simulink model "Ardupilot_PID_4"  (R2022a)
settings: Solver=VariableStepAuto  StartTime=0.0  StopTime=20.0  RelTol=1e-3
InitFcn:
  | addpath([pwd '/../Modeling']);
undefined symbols (not defined in the file or in its folder): DiscIntNeverNeededParam
libraries: simulink x8
settings Model: Creator=rodri  LastModifiedBy=rodri

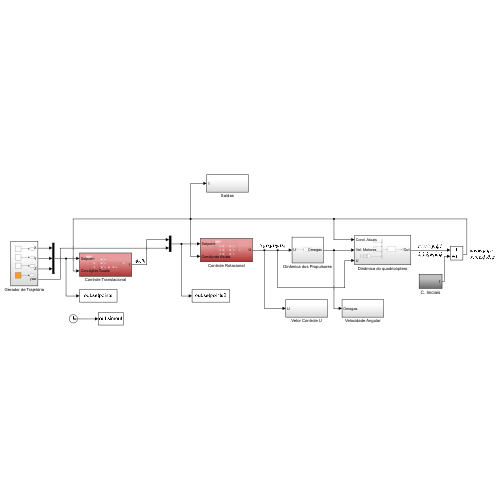
[thumbnail: Simulink's stored preview of the top-level diagram]
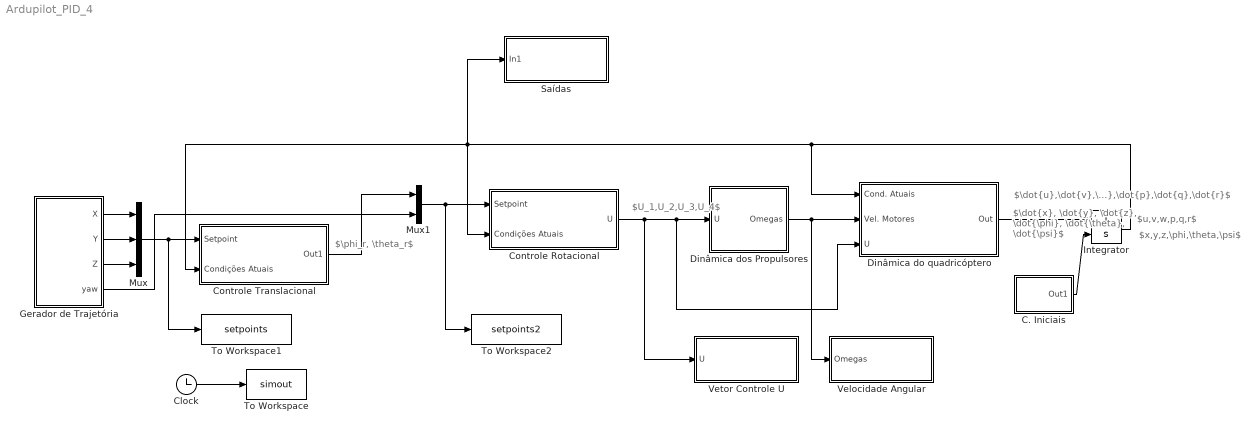
== system Ardupilot_PID_4 ==
  note: $x,y,z,\phi,\theta,\psi$
  note: $U_1,U_2,U_3,U_4$
  note: $u,v,w,p,q,r$
  note: $\phi_r, \theta_r$
  note: $\dot{u},\dot{v},\dot{w},\dot{p},\dot{q},\dot{r}$
  note: $\dot{x}, \dot{y}, \dot{z}, \dot{\phi}, \dot{\theta}, \dot{\psi}$
  C. Iniciais : Subsystem
  Clock : Clock
  Controle Rotacional : Subsystem
  Controle Translacional : Subsystem
  Dinâmica do quadricóptero : Subsystem
  Dinâmica dos Propulsores : Subsystem
  Gerador de Trajetória : Subsystem
  Integrator : Integrator  InitialConditionSource=external
  Mux : Mux  Inputs=3
  Mux1 : Mux  Inputs=2
  Saídas : Subsystem
  To Workspace : ToWorkspace  VariableName=simout  SaveFormat=Structure  SampleTime=-1
  To Workspace1 : ToWorkspace  VariableName=setpoints  SaveFormat=Timeseries  SampleTime=-1
  To Workspace2 : ToWorkspace  VariableName=setpoints2  SaveFormat=Timeseries  SampleTime=-1
  Velocidade Angular : Subsystem
  Vetor Controle U : Subsystem
  wires:
  Integrator/1 -> Dinâmica do quadricóptero/1(Cond. Atuais), Controle Rotacional/2(Condições Atuais), Saídas/1(In1), Controle Translacional/2(Condições Atuais)
  Dinâmica dos Propulsores/1(Omegas) -> Velocidade Angular/1(Omegas), Dinâmica do quadricóptero/2(Vel. Motores)
  Clock/1 -> To Workspace/1
  Controle Rotacional/1(U) -> Dinâmica do quadricóptero/3(U), Dinâmica dos Propulsores/1(U), Vetor Controle U/1(U)
  Mux/1 -> Controle Translacional/1(Setpoint), To Workspace1/1
  Dinâmica do quadricóptero/1(Out) -> Integrator/1
  Gerador de Trajetória/2(Y) -> Mux/2
  Controle Translacional/1(Out1) -> Mux1/1
  Gerador de Trajetória/3(Z) -> Mux/3
  Gerador de Trajetória/4(yaw) -> Mux1/2
  Mux1/1 -> To Workspace2/1, Controle Rotacional/1(Setpoint)
  Gerador de Trajetória/1(X) -> Mux/1
  C. Iniciais/1(Out1) -> Integrator/2

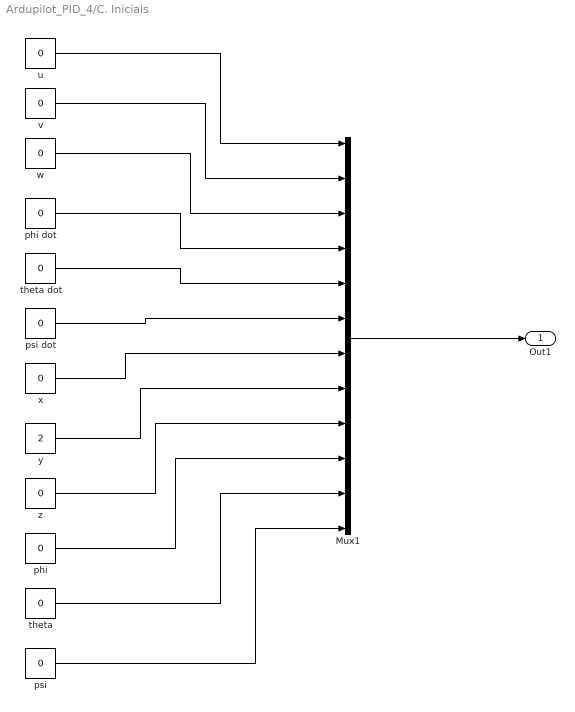
== system Ardupilot_PID_4/C. Iniciais ==
  Mux1 : Mux  Inputs=12
  phi : Constant  Value=0
  phi dot : Constant  Value=0
  psi : Constant  Value=0
  psi dot : Constant  Value=0
  theta : Constant  Value=0
  theta dot : Constant  Value=0
  u : Constant  Value=0
  v : Constant  Value=0
  w : Constant  Value=0
  x : Constant  Value=0
  y : Constant  Value=2
  z : Constant  Value=0
  Out1 : Outport
  wires:
  u/1 -> Mux1/1
  v/1 -> Mux1/2
  w/1 -> Mux1/3
  phi dot/1 -> Mux1/4
  theta dot/1 -> Mux1/5
  psi dot/1 -> Mux1/6
  x/1 -> Mux1/7
  y/1 -> Mux1/8
  z/1 -> Mux1/9
  phi/1 -> Mux1/10
  theta/1 -> Mux1/11
  psi/1 -> Mux1/12
  Mux1/1 -> Out1/1

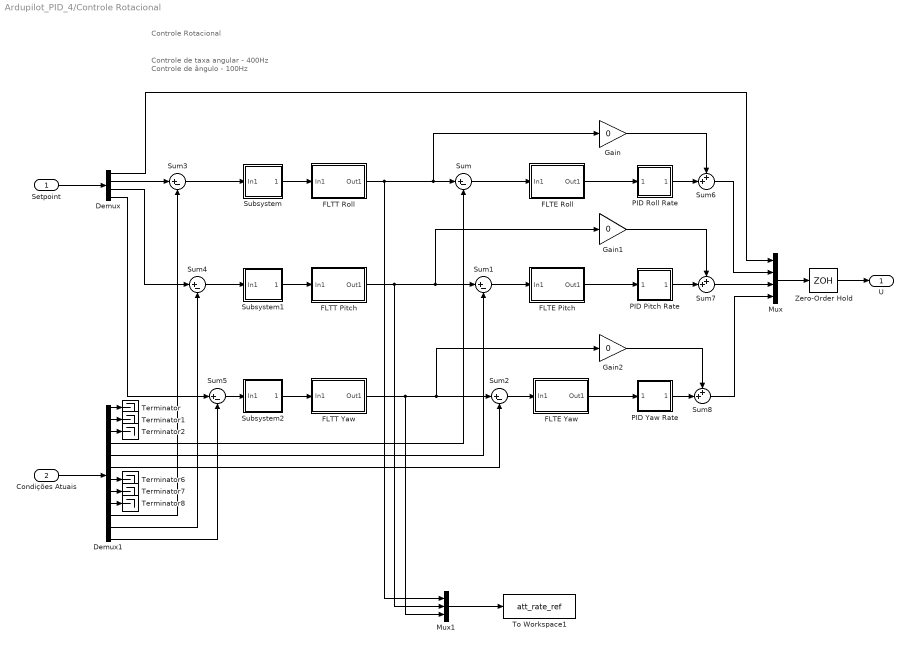
== system Ardupilot_PID_4/Controle Rotacional ==
  note: Controle de taxa angular - 400Hz
      | Controle de ângulo - 100Hz
  note: Controle Rotacional
  Setpoint : Inport
  Condições Atuais : Inport  Port=2
  Demux : Demux
  Demux1 : Demux  Outputs=12
  FLTE Pitch : Subsystem
  FLTE Roll : Subsystem
  FLTE Yaw : Subsystem
  FLTT Pitch : Subsystem
  FLTT Roll : Subsystem
  FLTT Yaw : Subsystem
  Gain : Gain  Gain=0
  Gain1 : Gain  Gain=0
  Gain2 : Gain  Gain=0
  Mux : Mux
  Mux1 : Mux  Inputs=3
  PID Pitch Rate : Subsystem
  PID Roll Rate : Subsystem
  PID Yaw Rate : Subsystem
  Subsystem : Subsystem  TreatAsAtomicUnit=on  SystemSampleTime=1/100
      mask Display: image('C:\Users\rodri\OneDrive\Imagens\Captura de tela 2025-05-23 002649.PNG'); % Use "Edit Image" on toolstrip to change.
  Subsystem1 : Subsystem  TreatAsAtomicUnit=on  SystemSampleTime=1/100
      mask Display: image('C:\Users\rodri\OneDrive\Imagens\Captura de tela 2025-05-23 002649.PNG'); % Use "Edit Image" on toolstrip to change.
  Subsystem2 : Subsystem  TreatAsAtomicUnit=on  SystemSampleTime=1/100
      mask Display: image('C:\Users\rodri\OneDrive\Imagens\Captura de tela 2025-05-23 002649.PNG'); % Use "Edit Image" on toolstrip to change.
  Sum{,1..5} (6 alike) : Sum  Inputs=|+-
  Sum6 : Sum  Inputs=++|
  Sum7 : Sum  Inputs=++|
  Sum8 : Sum  Inputs=++|
  Terminator{,1..2,6..8} (6 alike) : Terminator
  To Workspace1 : ToWorkspace  VariableName=att_rate_ref  SaveFormat=Timeseries  SampleTime=-1
  Zero-Order Hold : ZeroOrderHold  SampleTime=1/1000
  U : Outport
  wires:
  Condições Atuais/1 -> Demux1/1
  Demux1/10 -> Sum3/2
  Demux1/12 -> Sum5/2
  Demux1/11 -> Sum4/2
  Setpoint/1 -> Demux/1
  Demux1/1 -> Terminator/1
  Demux1/2 -> Terminator1/1
  Demux1/3 -> Terminator2/1
  Demux1/4 -> Sum/2
  Demux1/5 -> Sum1/2
  Demux1/6 -> Sum2/2
  Demux1/7 -> Terminator6/1
  Demux1/8 -> Terminator7/1
  Demux1/9 -> Terminator8/1
  Demux/1 -> Mux/1
  Demux/2 -> Sum3/1
  Demux/3 -> Sum4/1
  Demux/4 -> Sum5/1
  PID Roll Rate/1(Out1) -> Sum6/2
  Gain/1 -> Sum6/1
  Gain1/1 -> Sum7/1
  PID Pitch Rate/1(Out1) -> Sum7/2
  PID Yaw Rate/1(Out1) -> Sum8/2
  Gain2/1 -> Sum8/1
  Mux/1 -> Zero-Order Hold/1
  Sum3/1 -> Subsystem/1(In1)
  Sum4/1 -> Subsystem1/1(In1)
  Sum5/1 -> Subsystem2/1(In1)
  Sum7/1 -> Mux/3
  Sum8/1 -> Mux/4
  Sum6/1 -> Mux/2
  Zero-Order Hold/1 -> U/1
  Sum2/1 -> FLTE Yaw/1(In1)
  Sum1/1 -> FLTE Pitch/1(In1)
  Sum/1 -> FLTE Roll/1(In1)
  FLTE Yaw/1(Out1) -> PID Yaw Rate/1(In1)
  FLTE Pitch/1(Out1) -> PID Pitch Rate/1(In1)
  FLTE Roll/1(Out1) -> PID Roll Rate/1(In1)
  Subsystem1/1(Out1) -> FLTT Pitch/1(In1)
  Subsystem2/1(Out1) -> FLTT Yaw/1(In1)
  Subsystem/1(Out1) -> FLTT Roll/1(In1)
  FLTT Roll/1(Out1) -> Mux1/1, Sum/1, Gain/1
  Mux1/1 -> To Workspace1/1
  FLTT Pitch/1(Out1) -> Mux1/2, Gain1/1, Sum1/1
  FLTT Yaw/1(Out1) -> Mux1/3, Gain2/1, Sum2/1

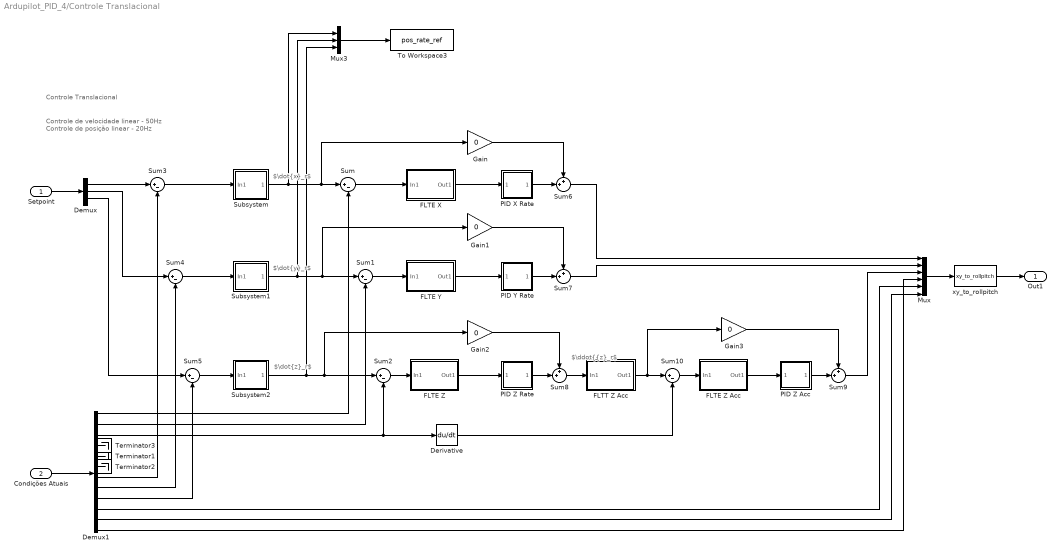
== system Ardupilot_PID_4/Controle Translacional ==
  note: $\dot{x}_r$
  note: $\dot{y}_r$
  note: Controle de velocidade linear - 50Hz
      | Controle de posição linear - 20Hz
  note: Controle Translacional
  note: $\dot{z}_r$
  note: $\ddot{{z}_r$
  Setpoint : Inport
  Condições Atuais : Inport  Port=2
  Demux : Demux  Outputs=3
  Demux1 : Demux  Outputs=12
  Derivative : Derivative
  FLTE X : Subsystem
  FLTE Y : Subsystem
  FLTE Z : Subsystem
  FLTE Z Acc : Subsystem
  FLTT Z Acc : Subsystem
  Gain{,1..3} (4 alike) : Gain  Gain=0
  Mux : Mux  Inputs=6
  Mux3 : Mux  Inputs=3
  PID X Rate : Subsystem
  PID Y Rate : Subsystem
  PID Z Acc : Subsystem
  PID Z Rate : Subsystem
  Subsystem : Subsystem  TreatAsAtomicUnit=on  SystemSampleTime=1/100
      mask Display: image('C:\Users\rodri\OneDrive\Imagens\Captura de tela 2025-05-23 002649.PNG'); % Use "Edit Image" on toolstrip to change.
  Subsystem1 : Subsystem  TreatAsAtomicUnit=on  SystemSampleTime=1/100
      mask Display: image('C:\Users\rodri\OneDrive\Imagens\Captura de tela 2025-05-23 002649.PNG'); % Use "Edit Image" on toolstrip to change.
  Subsystem2 : Subsystem  TreatAsAtomicUnit=on  SystemSampleTime=1/100
      mask Display: image('C:\Users\rodri\OneDrive\Imagens\Captura de tela 2025-05-23 002649.PNG'); % Use "Edit Image" on toolstrip to change.
  Sum{,1..5,10} (7 alike) : Sum  Inputs=|+-
  Sum{6..9} (4 alike) : Sum  Inputs=++|
  Terminator1 : Terminator
  Terminator2 : Terminator
  Terminator3 : Terminator
  To Workspace3 : ToWorkspace  VariableName=pos_rate_ref  SaveFormat=Timeseries  SampleTime=-1
  xy_to_rollpitch : MATLABFcn  MATLABFcn=xy_to_rollpitch  OutputDimensions=3
  Out1 : Outport
  wires:
  FLTE Y/1(Out1) -> PID Y Rate/1(In1)
  PID X Rate/1(Out1) -> Sum6/2
  FLTE X/1(Out1) -> PID X Rate/1(In1)
  FLTE Z/1(Out1) -> PID Z Rate/1(In1)
  Demux1/8 -> Sum4/2
  PID Y Rate/1(Out1) -> Sum7/2
  Setpoint/1 -> Demux/1
  Gain2/1 -> Sum8/1
  Sum/1 -> FLTE X/1(In1)
  Sum1/1 -> FLTE Y/1(In1)
  Sum7/1 -> Mux/2
  Sum4/1 -> Subsystem1/1(In1)
  Demux1/9 -> Sum5/2
  Demux1/1 -> Sum/2
  Sum3/1 -> Subsystem/1(In1)
  Gain1/1 -> Sum7/1
  Demux1/3 -> Derivative/1, Sum2/2
  Demux1/7 -> Sum3/2
  Mux/1 -> xy_to_rollpitch/1
  Gain/1 -> Sum6/1
  PID Z Rate/1(Out1) -> Sum8/2
  Condições Atuais/1 -> Demux1/1
  Demux1/2 -> Sum1/2
  Sum5/1 -> Subsystem2/1(In1)
  Sum6/1 -> Mux/1
  Sum2/1 -> FLTE Z/1(In1)
  Demux/1 -> Sum3/1
  Demux/2 -> Sum4/1
  Demux/3 -> Sum5/1
  xy_to_rollpitch/1 -> Out1/1
  Demux1/10 -> Mux/5
  Demux1/11 -> Mux/6
  Demux1/12 -> Mux/4
  FLTE Z Acc/1(Out1) -> PID Z Acc/1(In1)
  PID Z Acc/1(Out1) -> Sum9/2
  Sum8/1 -> FLTT Z Acc/1(In1)
  FLTT Z Acc/1(Out1) -> Gain3/1, Sum10/1
  Sum10/1 -> FLTE Z Acc/1(In1)
  Sum9/1 -> Mux/3
  Gain3/1 -> Sum9/1
  Derivative/1 -> Sum10/2
  Mux3/1 -> To Workspace3/1
  Subsystem/1(Out1) -> Mux3/1, Sum/1, Gain/1
  Subsystem2/1(Out1) -> Mux3/3, Gain2/1, Sum2/1
  Subsystem1/1(Out1) -> Gain1/1, Sum1/1, Mux3/2

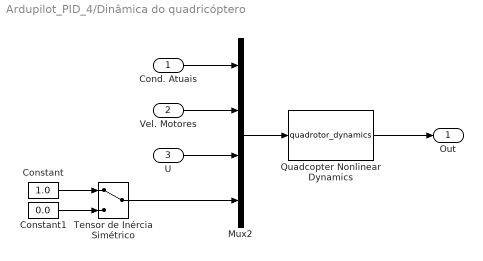
== system Ardupilot_PID_4/Dinâmica do quadricóptero ==
  Cond. Atuais : Inport
  Vel. Motores : Inport  Port=2
  U : Inport  Port=3
  Constant : Constant  Value=1.0
  Constant1 : Constant  Value=0.0
  Mux2 : Mux
  Quadcopter Nonlinear Dynamics : MATLABFcn  MATLABFcn=quadrotor_dynamics  OutputDimensions=12  OutputSignalType=real
  Tensor de Inércia Simétrico : ManualSwitch
  Out : Outport
  wires:
  Vel. Motores/1 -> Mux2/2
  Constant1/1 -> Tensor de Inércia Simétrico/2
  Mux2/1 -> Quadcopter Nonlinear Dynamics/1
  Constant/1 -> Tensor de Inércia Simétrico/1
  Quadcopter Nonlinear Dynamics/1 -> Out/1
  Cond. Atuais/1 -> Mux2/1
  Tensor de Inércia Simétrico/1 -> Mux2/4
  U/1 -> Mux2/3

== system Ardupilot_PID_4/Dinâmica dos Propulsores ==
  U : Inport
  Rotor Dynamics : MATLABFcn  MATLABFcn=rotor_dynamics  OutputDimensions=4  OutputSignalType=real
  Omegas : Outport
  wires:
  U/1 -> Rotor Dynamics/1
  Rotor Dynamics/1 -> Omegas/1

== system Ardupilot_PID_4/Gerador de Trajetória ==
  X signal : Sin  Amplitude=2  Frequency=2*pi/10  SampleTime=0
  Y signal : Sin  Amplitude=2  Frequency=2*pi/10  Phase=pi/2  SampleTime=0
  Yaw signal : Constant  Value=0
  Z signal : simulink/Sources/Ramp  slope=0.3  start=0  InitialOutput=0
  X : Outport
  Y : Outport  Port=2
  Z : Outport  Port=3
  yaw : Outport  Port=4
  wires:
  X signal/1 -> X/1
  Y signal/1 -> Y/1
  Yaw signal/1 -> yaw/1
  Z signal/1 -> Z/1

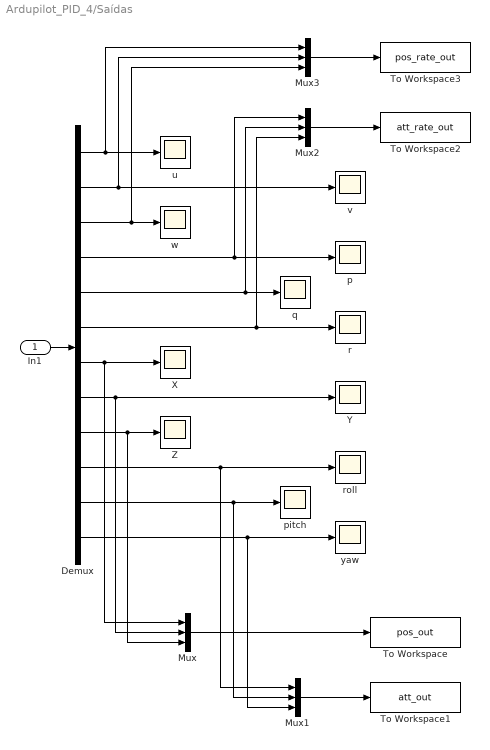
== system Ardupilot_PID_4/Saídas ==
  In1 : Inport
  Demux : Demux  Outputs=12
  Mux{,1..3} (4 alike) : Mux  Inputs=3
  To Workspace : ToWorkspace  VariableName=pos_out  SaveFormat=Timeseries  SampleTime=-1
  To Workspace1 : ToWorkspace  VariableName=att_out  SaveFormat=Timeseries  SampleTime=-1
  To Workspace2 : ToWorkspace  VariableName=att_rate_out  SaveFormat=Timeseries  SampleTime=-1
  To Workspace3 : ToWorkspace  VariableName=pos_rate_out  SaveFormat=Timeseries  SampleTime=-1
  X : Scope
  Y : Scope
  Z : Scope
  p : Scope
  pitch : Scope
  q : Scope
  r : Scope
  roll : Scope
  u : Scope
  v : Scope
  w : Scope
  yaw : Scope
  wires:
  In1/1 -> Demux/1
  Demux/1 -> Mux3/1, u/1
  Demux/2 -> Mux3/2, v/1
  Demux/3 -> Mux3/3, w/1
  Demux/4 -> Mux2/1, p/1
  Demux/5 -> Mux2/2, q/1
  Demux/6 -> Mux2/3, r/1
  Demux/7 -> X/1, Mux/1
  Demux/8 -> Mux/2, Y/1
  Demux/10 -> Mux1/1, roll/1
  Demux/11 -> Mux1/2, pitch/1
  Mux/1 -> To Workspace/1
  Mux1/1 -> To Workspace1/1
  Demux/12 -> Mux1/3, yaw/1
  Demux/9 -> Z/1, Mux/3
  Mux2/1 -> To Workspace2/1
  Mux3/1 -> To Workspace3/1

== system Ardupilot_PID_4/Velocidade Angular ==
  Omegas : Inport
  Demux : Demux
  Omega {1..4} (4 alike) : Scope
  To Workspace : ToWorkspace  VariableName=omegas  SaveFormat=Timeseries  SampleTime=-1
  wires:
  Demux/4 -> Omega 4/1
  Demux/3 -> Omega 3/1
  Demux/2 -> Omega 2/1
  Demux/1 -> Omega 1/1
  Omegas/1 -> To Workspace/1, Demux/1

== system Ardupilot_PID_4/Vetor Controle U ==
  U : Inport
  Demux : Demux
  To Workspace : ToWorkspace  VariableName=U  SaveFormat=Timeseries  SampleTime=-1
  U{1..4} (4 alike) : Scope
  wires:
  U/1 -> To Workspace/1, Demux/1
  Demux/1 -> U1/1
  Demux/2 -> U2/1
  Demux/3 -> U3/1
  Demux/4 -> U4/1

== system Ardupilot_PID_4/Controle Rotacional/FLTE Pitch ==
  In1 : Inport
  Constant : Constant
  Constant1 : Constant  Value=0
  Delay : Delay  DelayLength=1  InitialCondition=0
  Product : Product
  Product1 : Product
  Sum : Sum  Inputs=|++
  Out1 : Outport
  wires:
  Product/1 -> Sum/1
  In1/1 -> Product/1
  Constant/1 -> Product/2
  Sum/1 -> Out1/1, Delay/1
  Delay/1 -> Product1/1
  Product1/1 -> Sum/2
  Constant1/1 -> Product1/2

== system Ardupilot_PID_4/Controle Rotacional/FLTE Roll ==
  In1 : Inport
  Constant : Constant
  Constant1 : Constant  Value=0
  Delay : Delay  DelayLength=1  InitialCondition=0
  Product : Product
  Product1 : Product
  Sum : Sum  Inputs=|++
  Out1 : Outport
  wires:
  Product/1 -> Sum/1
  In1/1 -> Product/1
  Constant/1 -> Product/2
  Sum/1 -> Out1/1, Delay/1
  Delay/1 -> Product1/1
  Product1/1 -> Sum/2
  Constant1/1 -> Product1/2

== system Ardupilot_PID_4/Controle Rotacional/FLTE Yaw ==
  In1 : Inport
  Constant : Constant  Value=0.0385
  Constant1 : Constant  Value=0.9615
  Delay : Delay  DelayLength=1  InitialCondition=0
  Product : Product
  Product1 : Product
  Sum : Sum  Inputs=|++
  Out1 : Outport
  wires:
  Product/1 -> Sum/1
  In1/1 -> Product/1
  Constant/1 -> Product/2
  Sum/1 -> Out1/1, Delay/1
  Delay/1 -> Product1/1
  Product1/1 -> Sum/2
  Constant1/1 -> Product1/2

== system Ardupilot_PID_4/Controle Rotacional/FLTT Pitch ==
  In1 : Inport
  Constant : Constant  Value=0.2696
  Constant1 : Constant  Value=0.7304
  Delay : Delay  DelayLength=1  InitialCondition=0
  Product : Product
  Product1 : Product
  Sum : Sum  Inputs=|++
  Out1 : Outport
  wires:
  Product/1 -> Sum/1
  In1/1 -> Product/1
  Constant/1 -> Product/2
  Sum/1 -> Out1/1, Delay/1
  Delay/1 -> Product1/1
  Product1/1 -> Sum/2
  Constant1/1 -> Product1/2

== system Ardupilot_PID_4/Controle Rotacional/FLTT Roll ==
  note: $\alpha$
  note: $1-\alpha$
  In1 : Inport
  Constant : Constant  Value=0.2696
  Constant1 : Constant  Value=0.7304
  Delay : Delay  DelayLength=1  InitialCondition=0
  Product : Product
  Product1 : Product
  Sum : Sum  Inputs=|++
  Out1 : Outport
  wires:
  Product/1 -> Sum/1
  In1/1 -> Product/1
  Constant/1 -> Product/2
  Sum/1 -> Out1/1, Delay/1
  Delay/1 -> Product1/1
  Product1/1 -> Sum/2
  Constant1/1 -> Product1/2

== system Ardupilot_PID_4/Controle Rotacional/FLTT Yaw ==
  In1 : Inport
  Constant : Constant  Value=0.2696
  Constant1 : Constant  Value=0.7304
  Delay : Delay  DelayLength=1  InitialCondition=0
  Product : Product
  Product1 : Product
  Sum : Sum  Inputs=|++
  Out1 : Outport
  wires:
  Product/1 -> Sum/1
  In1/1 -> Product/1
  Constant/1 -> Product/2
  Sum/1 -> Out1/1, Delay/1
  Delay/1 -> Product1/1
  Product1/1 -> Sum/2
  Constant1/1 -> Product1/2

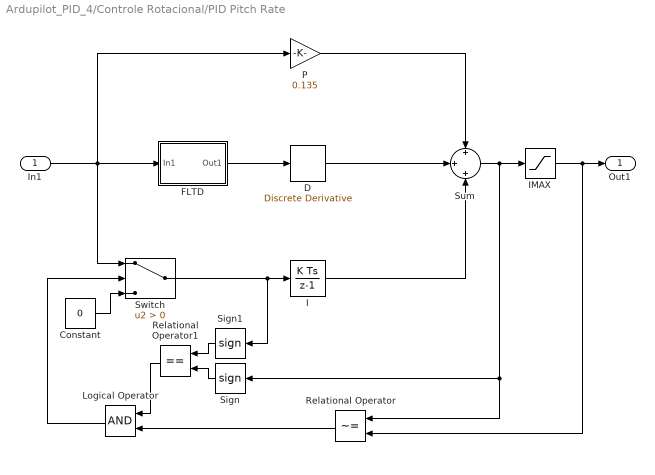
== system Ardupilot_PID_4/Controle Rotacional/PID Pitch Rate ==
  In1 : Inport
  Constant : Constant  Value=0
  D : simulink/Discrete/Discrete Derivative  gainval=0.0036  ICPrevScaledInput=0.0  OutMin=[]  OutMax=[]  OutDataType=fixdt(1, 16)  OutScaling=2^-10  DoSatur=off
  FLTD : Subsystem
  I : DiscreteIntegrator  gainval=0.135  SampleTime=-1  ICPrevOutput=DiscIntNeverNeededParam  ICPrevScaledInput=DiscIntNeverNeededParam
  IMAX : Saturate
  Logical Operator : Logic  AllPortsSameDT=off  OutDataTypeStr=boolean
  P : Gain  Gain=0.135
  Relational Operator : RelationalOperator  Operator=~=  OutDataTypeStr=boolean  RndMeth=Simplest  InputSameDT=off
  Relational Operator1 : RelationalOperator  Operator===  OutDataTypeStr=boolean  RndMeth=Simplest  InputSameDT=off
  Sign : Signum
  Sign1 : Signum
  Sum : Sum  Inputs=+|+|+
  Switch : Switch  Criteria=u2 > Threshold  SaturateOnIntegerOverflow=off  InputSameDT=off
  Out1 : Outport
  wires:
  D/1 -> Sum/2
  P/1 -> Sum/1
  FLTD/1(Out1) -> D/1
  Logical Operator/1 -> Switch/2
  Relational Operator1/1 -> Logical Operator/1
  Constant/1 -> Switch/3
  Relational Operator/1 -> Logical Operator/2
  Sign1/1 -> Relational Operator1/1
  Switch/1 -> Sign1/1, I/1
  In1/1 -> Switch/1, FLTD/1(In1), P/1
  I/1 -> Sum/3
  Sign/1 -> Relational Operator1/2
  IMAX/1 -> Relational Operator/2, Out1/1
  Sum/1 -> Sign/1, Relational Operator/1, IMAX/1

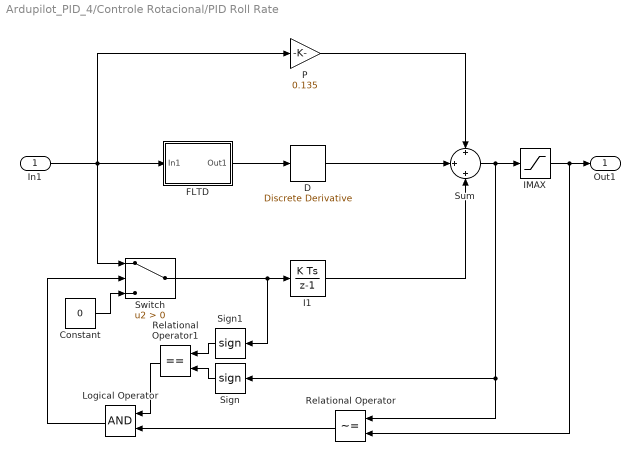
== system Ardupilot_PID_4/Controle Rotacional/PID Roll Rate ==
  In1 : Inport
  Constant : Constant  Value=0
  D : simulink/Discrete/Discrete Derivative  gainval=0.0036  ICPrevScaledInput=0.0  OutMin=[]  OutMax=[]  OutDataType=fixdt(1, 16)  OutScaling=2^-10  DoSatur=off
  FLTD : Subsystem
  I1 : DiscreteIntegrator  gainval=0.135  SampleTime=-1  ICPrevOutput=DiscIntNeverNeededParam  ICPrevScaledInput=DiscIntNeverNeededParam
  IMAX : Saturate
  Logical Operator : Logic  AllPortsSameDT=off  OutDataTypeStr=boolean
  P : Gain  Gain=0.135
  Relational Operator : RelationalOperator  Operator=~=  OutDataTypeStr=boolean  RndMeth=Simplest  InputSameDT=off
  Relational Operator1 : RelationalOperator  Operator===  OutDataTypeStr=boolean  RndMeth=Simplest  InputSameDT=off
  Sign : Signum
  Sign1 : Signum
  Sum : Sum  Inputs=+|+|+
  Switch : Switch  Criteria=u2 > Threshold  SaturateOnIntegerOverflow=off  InputSameDT=off
  Out1 : Outport
  wires:
  D/1 -> Sum/2
  P/1 -> Sum/1
  FLTD/1(Out1) -> D/1
  Logical Operator/1 -> Switch/2
  Relational Operator1/1 -> Logical Operator/1
  Constant/1 -> Switch/3
  Relational Operator/1 -> Logical Operator/2
  Sign1/1 -> Relational Operator1/1
  Switch/1 -> Sign1/1, I1/1
  In1/1 -> Switch/1, FLTD/1(In1), P/1
  I1/1 -> Sum/3
  Sign/1 -> Relational Operator1/2
  IMAX/1 -> Relational Operator/2, Out1/1
  Sum/1 -> Relational Operator/1, Sign/1, IMAX/1

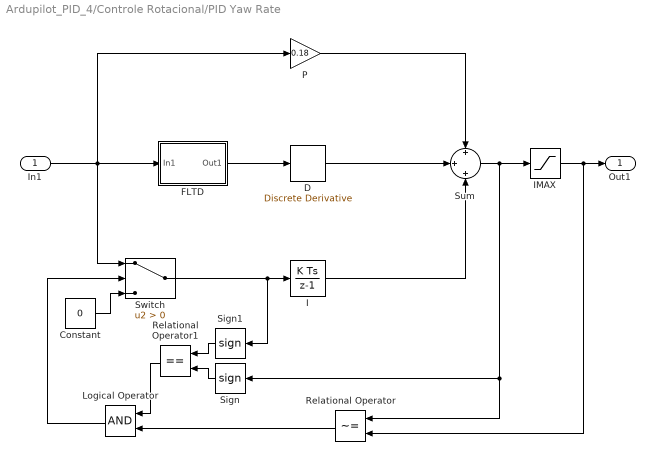
== system Ardupilot_PID_4/Controle Rotacional/PID Yaw Rate ==
  In1 : Inport
  Constant : Constant  Value=0
  D : simulink/Discrete/Discrete Derivative  gainval=0  ICPrevScaledInput=0.0  OutMin=[]  OutMax=[]  OutDataType=fixdt(1, 16)  OutScaling=2^-10  DoSatur=off
  FLTD : Subsystem
  I : DiscreteIntegrator  gainval=0.018  SampleTime=-1  ICPrevOutput=DiscIntNeverNeededParam  ICPrevScaledInput=DiscIntNeverNeededParam
  IMAX : Saturate
  Logical Operator : Logic  AllPortsSameDT=off  OutDataTypeStr=boolean
  P : Gain  Gain=0.18
  Relational Operator : RelationalOperator  Operator=~=  OutDataTypeStr=boolean  RndMeth=Simplest  InputSameDT=off
  Relational Operator1 : RelationalOperator  Operator===  OutDataTypeStr=boolean  RndMeth=Simplest  InputSameDT=off
  Sign : Signum
  Sign1 : Signum
  Sum : Sum  Inputs=+|+|+
  Switch : Switch  Criteria=u2 > Threshold  SaturateOnIntegerOverflow=off  InputSameDT=off
  Out1 : Outport
  wires:
  D/1 -> Sum/2
  P/1 -> Sum/1
  FLTD/1(Out1) -> D/1
  Constant/1 -> Switch/3
  Sign/1 -> Relational Operator1/2
  Sign1/1 -> Relational Operator1/1
  Relational Operator1/1 -> Logical Operator/1
  Switch/1 -> Sign1/1, I/1
  Logical Operator/1 -> Switch/2
  Sum/1 -> Sign/1, Relational Operator/1, IMAX/1
  In1/1 -> Switch/1, FLTD/1(In1), P/1
  I/1 -> Sum/3
  Relational Operator/1 -> Logical Operator/2
  IMAX/1 -> Relational Operator/2, Out1/1

== system Ardupilot_PID_4/Controle Rotacional/Subsystem ==
  note: a max
  note: Kp
  In1 : Inport
  Constant : Constant  Value=4.5
  Constant1 : Constant  Value=19.19
  Interpreted MATLAB Function : MATLABFcn  MATLABFcn=sqrt_controller
  Mux : Mux  Inputs=3
  Out1 : Outport
  wires:
  In1/1 -> Mux/1
  Constant/1 -> Mux/2
  Constant1/1 -> Mux/3
  Mux/1 -> Interpreted MATLAB Function/1
  Interpreted MATLAB Function/1 -> Out1/1

== system Ardupilot_PID_4/Controle Rotacional/Subsystem1 ==
  note: Kp
  note: a max
  In1 : Inport
  Constant : Constant  Value=4.5
  Constant1 : Constant  Value=19.19
  Interpreted MATLAB Function : MATLABFcn  MATLABFcn=sqrt_controller
  Mux : Mux  Inputs=3
  Out1 : Outport
  wires:
  In1/1 -> Mux/1
  Constant/1 -> Mux/2
  Constant1/1 -> Mux/3
  Mux/1 -> Interpreted MATLAB Function/1
  Interpreted MATLAB Function/1 -> Out1/1

== system Ardupilot_PID_4/Controle Rotacional/Subsystem2 ==
  note: Kp
  note: a max
  In1 : Inport
  Constant : Constant  Value=4.5
  Constant1 : Constant  Value=4.71
  Interpreted MATLAB Function : MATLABFcn  MATLABFcn=sqrt_controller
  Mux : Mux  Inputs=3
  Out1 : Outport
  wires:
  In1/1 -> Mux/1
  Constant/1 -> Mux/2
  Constant1/1 -> Mux/3
  Mux/1 -> Interpreted MATLAB Function/1
  Interpreted MATLAB Function/1 -> Out1/1

== system Ardupilot_PID_4/Controle Translacional/FLTE X ==
  In1 : Inport
  Constant : Constant  Value=0.4665
  Constant1 : Constant  Value=0.5335
  Delay : Delay  DelayLength=1  InitialCondition=0
  Product : Product
  Product1 : Product
  Sum : Sum  Inputs=|++
  Out1 : Outport
  wires:
  Product/1 -> Sum/1
  In1/1 -> Product/1
  Constant/1 -> Product/2
  Sum/1 -> Out1/1, Delay/1
  Delay/1 -> Product1/1
  Product1/1 -> Sum/2
  Constant1/1 -> Product1/2

== system Ardupilot_PID_4/Controle Translacional/FLTE Y ==
  In1 : Inport
  Constant : Constant  Value=0.4665
  Constant1 : Constant  Value=0.5335
  Delay : Delay  DelayLength=1  InitialCondition=0
  Product : Product
  Product1 : Product
  Sum : Sum  Inputs=|++
  Out1 : Outport
  wires:
  Product/1 -> Sum/1
  In1/1 -> Product/1
  Constant/1 -> Product/2
  Sum/1 -> Out1/1, Delay/1
  Delay/1 -> Product1/1
  Product1/1 -> Sum/2
  Constant1/1 -> Product1/2

== system Ardupilot_PID_4/Controle Translacional/FLTE Z ==
  In1 : Inport
  Constant : Constant  Value=0.4665
  Constant1 : Constant  Value=0.5535
  Delay : Delay  DelayLength=1  InitialCondition=0
  Product : Product
  Product1 : Product
  Sum : Sum  Inputs=|++
  Out1 : Outport
  wires:
  Product/1 -> Sum/1
  In1/1 -> Product/1
  Constant/1 -> Product/2
  Sum/1 -> Out1/1, Delay/1
  Delay/1 -> Product1/1
  Product1/1 -> Sum/2
  Constant1/1 -> Product1/2

== system Ardupilot_PID_4/Controle Translacional/FLTE Z Acc ==
  In1 : Inport
  Constant : Constant  Value=0.9189
  Constant1 : Constant  Value=0.0811
  Delay : Delay  DelayLength=1  InitialCondition=0
  Product : Product
  Product1 : Product
  Sum : Sum  Inputs=|++
  Out1 : Outport
  wires:
  Product/1 -> Sum/1
  In1/1 -> Product/1
  Constant/1 -> Product/2
  Sum/1 -> Out1/1, Delay/1
  Delay/1 -> Product1/1
  Product1/1 -> Sum/2
  Constant1/1 -> Product1/2

== system Ardupilot_PID_4/Controle Translacional/FLTT Z Acc ==
  In1 : Inport
  Constant : Constant
  Constant1 : Constant  Value=0
  Delay : Delay  DelayLength=1  InitialCondition=0
  Product : Product
  Product1 : Product
  Sum : Sum  Inputs=|++
  Out1 : Outport
  wires:
  Product/1 -> Sum/1
  In1/1 -> Product/1
  Constant/1 -> Product/2
  Sum/1 -> Out1/1, Delay/1
  Delay/1 -> Product1/1
  Product1/1 -> Sum/2
  Constant1/1 -> Product1/2

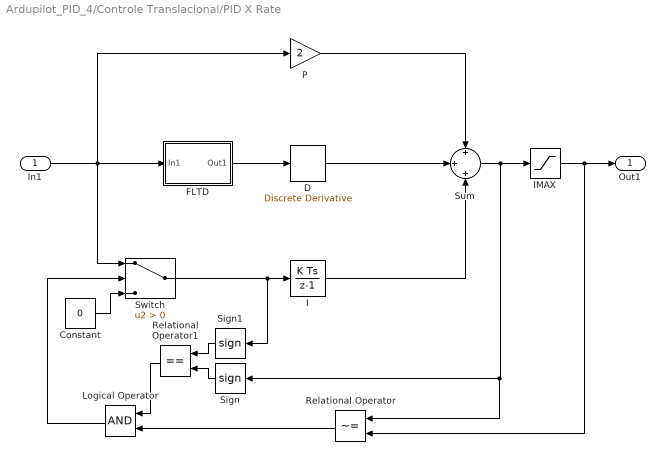
== system Ardupilot_PID_4/Controle Translacional/PID X Rate ==
  In1 : Inport
  Constant : Constant  Value=0
  D : simulink/Discrete/Discrete Derivative  gainval=0.5  ICPrevScaledInput=0.0  OutMin=[]  OutMax=[]  OutDataType=fixdt(1, 16)  OutScaling=2^-10  DoSatur=off
  FLTD : Subsystem
  I : DiscreteIntegrator  gainval=1  SampleTime=-1  ICPrevOutput=DiscIntNeverNeededParam  ICPrevScaledInput=DiscIntNeverNeededParam
  IMAX : Saturate  UpperLimit=10  LowerLimit=-10
  Logical Operator : Logic  AllPortsSameDT=off  OutDataTypeStr=boolean
  P : Gain  Gain=2
  Relational Operator : RelationalOperator  Operator=~=  OutDataTypeStr=boolean  RndMeth=Simplest  InputSameDT=off
  Relational Operator1 : RelationalOperator  Operator===  OutDataTypeStr=boolean  RndMeth=Simplest  InputSameDT=off
  Sign : Signum
  Sign1 : Signum
  Sum : Sum  Inputs=+|+|+
  Switch : Switch  Criteria=u2 > Threshold  SaturateOnIntegerOverflow=off  InputSameDT=off
  Out1 : Outport
  wires:
  D/1 -> Sum/2
  P/1 -> Sum/1
  FLTD/1(Out1) -> D/1
  Sum/1 -> Sign/1, Relational Operator/1, IMAX/1
  Switch/1 -> Sign1/1, I/1
  Sign/1 -> Relational Operator1/2
  Relational Operator1/1 -> Logical Operator/1
  Logical Operator/1 -> Switch/2
  Relational Operator/1 -> Logical Operator/2
  Constant/1 -> Switch/3
  In1/1 -> Switch/1, FLTD/1(In1), P/1
  Sign1/1 -> Relational Operator1/1
  I/1 -> Sum/3
  IMAX/1 -> Relational Operator/2, Out1/1

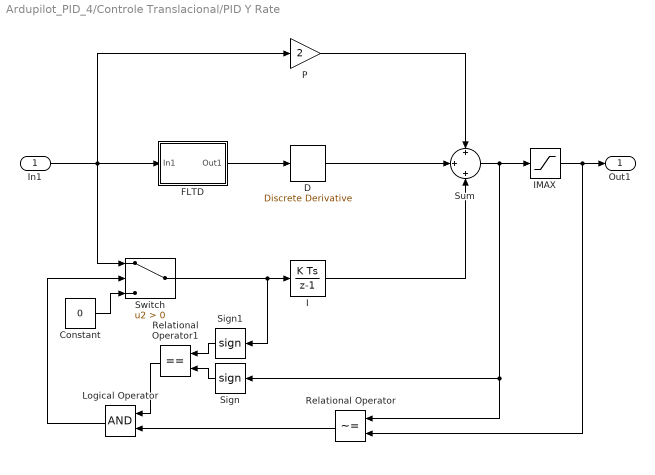
== system Ardupilot_PID_4/Controle Translacional/PID Y Rate ==
  In1 : Inport
  Constant : Constant  Value=0
  D : simulink/Discrete/Discrete Derivative  gainval=0.5  ICPrevScaledInput=0.0  OutMin=[]  OutMax=[]  OutDataType=fixdt(1, 16)  OutScaling=2^-10  DoSatur=off
  FLTD : Subsystem
  I : DiscreteIntegrator  gainval=1  SampleTime=-1  ICPrevOutput=DiscIntNeverNeededParam  ICPrevScaledInput=DiscIntNeverNeededParam
  IMAX : Saturate  UpperLimit=10  LowerLimit=-10
  Logical Operator : Logic  AllPortsSameDT=off  OutDataTypeStr=boolean
  P : Gain  Gain=2
  Relational Operator : RelationalOperator  Operator=~=  OutDataTypeStr=boolean  RndMeth=Simplest  InputSameDT=off
  Relational Operator1 : RelationalOperator  Operator===  OutDataTypeStr=boolean  RndMeth=Simplest  InputSameDT=off
  Sign : Signum
  Sign1 : Signum
  Sum : Sum  Inputs=+|+|+
  Switch : Switch  Criteria=u2 > Threshold  SaturateOnIntegerOverflow=off  InputSameDT=off
  Out1 : Outport
  wires:
  D/1 -> Sum/2
  P/1 -> Sum/1
  FLTD/1(Out1) -> D/1
  In1/1 -> Switch/1, FLTD/1(In1), P/1
  Sign1/1 -> Relational Operator1/1
  Constant/1 -> Switch/3
  Relational Operator/1 -> Logical Operator/2
  Relational Operator1/1 -> Logical Operator/1
  Logical Operator/1 -> Switch/2
  Sum/1 -> Sign/1, Relational Operator/1, IMAX/1
  I/1 -> Sum/3
  Switch/1 -> Sign1/1, I/1
  Sign/1 -> Relational Operator1/2
  IMAX/1 -> Relational Operator/2, Out1/1

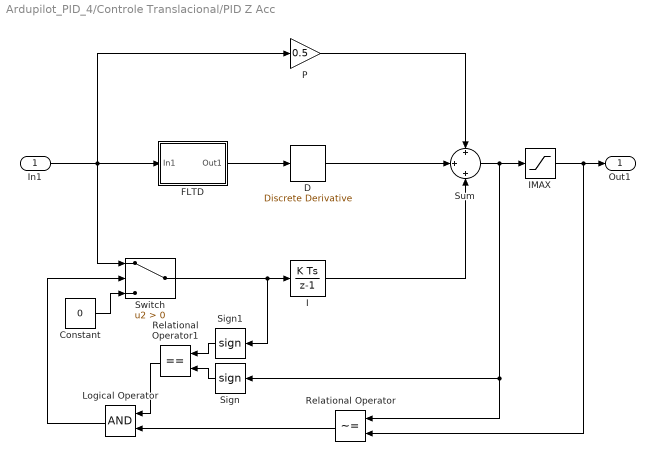
== system Ardupilot_PID_4/Controle Translacional/PID Z Acc ==
  In1 : Inport
  Constant : Constant  Value=0
  D : simulink/Discrete/Discrete Derivative  gainval=0  ICPrevScaledInput=0.0  OutMin=[]  OutMax=[]  OutDataType=fixdt(1, 16)  OutScaling=2^-10  DoSatur=off
  FLTD : Subsystem
  I : DiscreteIntegrator  gainval=1  SampleTime=-1  ICPrevOutput=DiscIntNeverNeededParam  ICPrevScaledInput=DiscIntNeverNeededParam
  IMAX : Saturate  UpperLimit=80  LowerLimit=-80
  Logical Operator : Logic  AllPortsSameDT=off  OutDataTypeStr=boolean
  P : Gain  Gain=0.5
  Relational Operator : RelationalOperator  Operator=~=  OutDataTypeStr=boolean  RndMeth=Simplest  InputSameDT=off
  Relational Operator1 : RelationalOperator  Operator===  OutDataTypeStr=boolean  RndMeth=Simplest  InputSameDT=off
  Sign : Signum
  Sign1 : Signum
  Sum : Sum  Inputs=+|+|+
  Switch : Switch  Criteria=u2 > Threshold  SaturateOnIntegerOverflow=off  InputSameDT=off
  Out1 : Outport
  wires:
  D/1 -> Sum/2
  P/1 -> Sum/1
  FLTD/1(Out1) -> D/1
  Relational Operator/1 -> Logical Operator/2
  Relational Operator1/1 -> Logical Operator/1
  Sign/1 -> Relational Operator1/2
  Logical Operator/1 -> Switch/2
  Sign1/1 -> Relational Operator1/1
  Switch/1 -> Sign1/1, I/1
  Constant/1 -> Switch/3
  Sum/1 -> Sign/1, Relational Operator/1, IMAX/1
  I/1 -> Sum/3
  In1/1 -> Switch/1, FLTD/1(In1), P/1
  IMAX/1 -> Relational Operator/2, Out1/1

== system Ardupilot_PID_4/Controle Translacional/PID Z Rate ==
  In1 : Inport
  D : simulink/Discrete/Discrete Derivative  gainval=0  ICPrevScaledInput=0.0  OutMin=[]  OutMax=[]  OutDataType=fixdt(1, 16)  OutScaling=2^-10  DoSatur=off
  FLTD : Subsystem
  P : Gain  Gain=5
  Sum : Sum  Inputs=++|
  Out1 : Outport
  wires:
  In1/1 -> FLTD/1(In1), P/1
  Sum/1 -> Out1/1
  P/1 -> Sum/1
  FLTD/1(Out1) -> D/1
  D/1 -> Sum/2

== system Ardupilot_PID_4/Controle Translacional/Subsystem ==
  note: a max
  note: Kp
  In1 : Inport
  Constant : Constant
  Constant1 : Constant  Value=5
  Interpreted MATLAB Function : MATLABFcn  MATLABFcn=sqrt_controller
  Mux : Mux  Inputs=3
  Out1 : Outport
  wires:
  In1/1 -> Mux/1
  Constant/1 -> Mux/2
  Constant1/1 -> Mux/3
  Mux/1 -> Interpreted MATLAB Function/1
  Interpreted MATLAB Function/1 -> Out1/1

== system Ardupilot_PID_4/Controle Translacional/Subsystem1 ==
  note: Kp
  note: a max
  In1 : Inport
  Constant : Constant
  Constant1 : Constant  Value=5
  Interpreted MATLAB Function : MATLABFcn  MATLABFcn=sqrt_controller
  Mux : Mux  Inputs=3
  Out1 : Outport
  wires:
  In1/1 -> Mux/1
  Constant/1 -> Mux/2
  Constant1/1 -> Mux/3
  Mux/1 -> Interpreted MATLAB Function/1
  Interpreted MATLAB Function/1 -> Out1/1

== system Ardupilot_PID_4/Controle Translacional/Subsystem2 ==
  note: Kp
  note: a max
  In1 : Inport
  Constant : Constant
  Constant1 : Constant
  Interpreted MATLAB Function : MATLABFcn  MATLABFcn=sqrt_controller
  Mux : Mux  Inputs=3
  Out1 : Outport
  wires:
  In1/1 -> Mux/1
  Constant/1 -> Mux/2
  Constant1/1 -> Mux/3
  Mux/1 -> Interpreted MATLAB Function/1
  Interpreted MATLAB Function/1 -> Out1/1

== system Ardupilot_PID_4/Controle Rotacional/PID Pitch Rate/FLTD ==
  In1 : Inport
  Constant : Constant  Value=0.2696
  Constant1 : Constant  Value=0.7304
  Delay : Delay  DelayLength=1  InitialCondition=0
  Product : Product
  Product1 : Product
  Sum : Sum  Inputs=|++
  Out1 : Outport
  wires:
  Product/1 -> Sum/1
  In1/1 -> Product/1
  Constant/1 -> Product/2
  Sum/1 -> Out1/1, Delay/1
  Delay/1 -> Product1/1
  Product1/1 -> Sum/2
  Constant1/1 -> Product1/2

== system Ardupilot_PID_4/Controle Rotacional/PID Roll Rate/FLTD ==
  In1 : Inport
  Constant : Constant  Value=0.2696
  Constant1 : Constant  Value=0.7304
  Delay : Delay  DelayLength=1  InitialCondition=0
  Product : Product
  Product1 : Product
  Sum : Sum  Inputs=|++
  Out1 : Outport
  wires:
  Product/1 -> Sum/1
  In1/1 -> Product/1
  Constant/1 -> Product/2
  Sum/1 -> Out1/1, Delay/1
  Delay/1 -> Product1/1
  Product1/1 -> Sum/2
  Constant1/1 -> Product1/2

== system Ardupilot_PID_4/Controle Rotacional/PID Yaw Rate/FLTD ==
  In1 : Inport
  Constant : Constant  Value=0.2696
  Constant1 : Constant  Value=0.7304
  Delay : Delay  DelayLength=1  InitialCondition=0
  Product : Product
  Product1 : Product
  Sum : Sum  Inputs=|++
  Out1 : Outport
  wires:
  Product/1 -> Sum/1
  In1/1 -> Product/1
  Constant/1 -> Product/2
  Sum/1 -> Out1/1, Delay/1
  Delay/1 -> Product1/1
  Product1/1 -> Sum/2
  Constant1/1 -> Product1/2

== system Ardupilot_PID_4/Controle Translacional/PID X Rate/FLTD ==
  In1 : Inport
  Constant : Constant  Value=0.4665
  Constant1 : Constant  Value=0.5335
  Delay : Delay  DelayLength=1  InitialCondition=0
  Product : Product
  Product1 : Product
  Sum : Sum  Inputs=|++
  Out1 : Outport
  wires:
  Product/1 -> Sum/1
  In1/1 -> Product/1
  Constant/1 -> Product/2
  Sum/1 -> Out1/1, Delay/1
  Delay/1 -> Product1/1
  Product1/1 -> Sum/2
  Constant1/1 -> Product1/2

== system Ardupilot_PID_4/Controle Translacional/PID Y Rate/FLTD ==
  In1 : Inport
  Constant : Constant  Value=0.4665
  Constant1 : Constant  Value=0.5335
  Delay : Delay  DelayLength=1  InitialCondition=0
  Product : Product
  Product1 : Product
  Sum : Sum  Inputs=|++
  Out1 : Outport
  wires:
  Product/1 -> Sum/1
  In1/1 -> Product/1
  Constant/1 -> Product/2
  Sum/1 -> Out1/1, Delay/1
  Delay/1 -> Product1/1
  Product1/1 -> Sum/2
  Constant1/1 -> Product1/2

== system Ardupilot_PID_4/Controle Translacional/PID Z Acc/FLTD ==
  In1 : Inport
  Constant : Constant
  Constant1 : Constant  Value=0
  Delay : Delay  DelayLength=1  InitialCondition=0
  Product : Product
  Product1 : Product
  Sum : Sum  Inputs=|++
  Out1 : Outport
  wires:
  Product/1 -> Sum/1
  In1/1 -> Product/1
  Constant/1 -> Product/2
  Sum/1 -> Out1/1, Delay/1
  Delay/1 -> Product1/1
  Product1/1 -> Sum/2
  Constant1/1 -> Product1/2

== system Ardupilot_PID_4/Controle Translacional/PID Z Rate/FLTD ==
  In1 : Inport
  Constant : Constant  Value=0.2696
  Constant1 : Constant  Value=0.7304
  Delay : Delay  DelayLength=1  InitialCondition=0
  Product : Product
  Product1 : Product
  Sum : Sum  Inputs=|++
  Out1 : Outport
  wires:
  Product/1 -> Sum/1
  In1/1 -> Product/1
  Constant/1 -> Product/2
  Sum/1 -> Out1/1, Delay/1
  Delay/1 -> Product1/1
  Product1/1 -> Sum/2
  Constant1/1 -> Product1/2
